simulink model "MQIF_Neuron"  (R2024b)
settings: Solver=ode1  StartTime=0.0  StopTime=10  FixedStep=1e-4  RelTol=1e-3
undefined symbols (not defined in the file): Vus0
settings Model: Creator=Serious Chimp  LastModifiedBy=31194
settings SolverCC: EnableFixedStepZeroCrossing=on
settings RTWCC: GPUComputeCapability=3.5

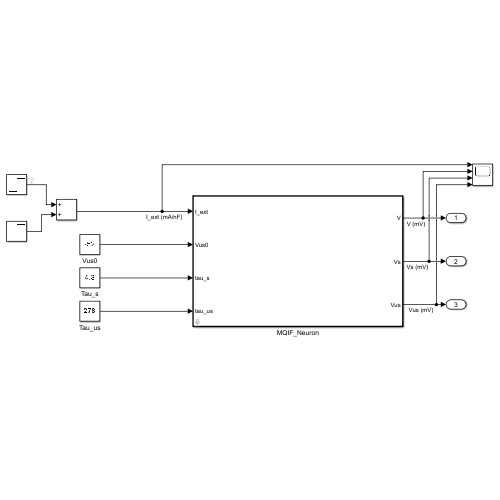
[thumbnail: Simulink's stored preview of the top-level diagram]
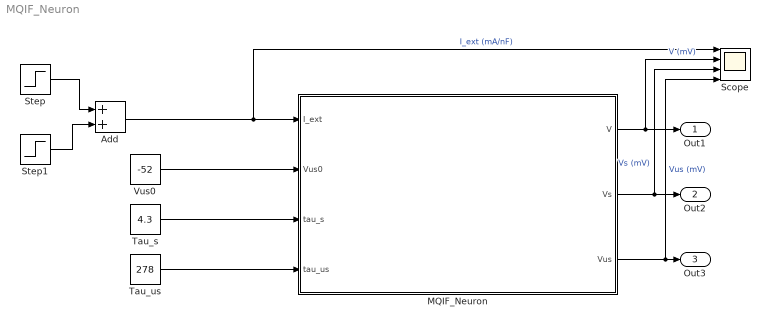
== system MQIF_Neuron ==
  Add : Sum
  MQIF_Neuron : Subsystem  TreatAsAtomicUnit=on  mask{V0=-52, Vs0=-50, V_threshold=20, V_reset=-45, Vs_reset=7.5, delta_Vus=1.7, g_f=1.0, g_s=0.5, g_us=0.015, C=0.82}
      mask prompts: V0 "Equilibrium V0"; Vs0 "Equilibrium Vs0"; V_threshold "Threshold for Spike, V_thresh"; V_reset "After-spike Reset Votlage, V_r"; Vs_reset "After-spike Reset Vs, Vs_r"; delta_Vus "Vus After-spike Memory, delta_Vus"; g_f "I Conductance, g_f"; g_s "I_us Conductance, g_s"; g_us "I_us Conductance, g_us"; C "Capacitance, C"
      mask DialogControl NeuronStateVariables Prompt: Parameters
  Scope : Scope  NumInputPorts=4
  Step : Step  After=5  SampleTime=0
  Step1 : Step  Time=0  After=0  SampleTime=0
  Tau_s : Constant  Value=4.3
  Tau_us : Constant  Value=278
  Vus0 : Constant  Value=-52
  Out1 : Outport
  Out2 : Outport  Port=2
  Out3 : Outport  Port=3
  wires:
  Add/1 -> Scope/1, MQIF_Neuron/1(I_ext)  "I_ext (mA/nF)"
  MQIF_Neuron/1(V) -> Scope/2, Out1/1  "V (mV)"
  MQIF_Neuron/2(Vs) -> Scope/3, Out2/1  "Vs (mV)"
  MQIF_Neuron/3(Vus) -> Scope/4, Out3/1  "Vus (mV)"
  Vus0/1 -> MQIF_Neuron/2(Vus0)
  Tau_s/1 -> MQIF_Neuron/3(tau_s)
  Tau_us/1 -> MQIF_Neuron/4(tau_us)
  Step/1 -> Add/1
  Step1/1 -> Add/2

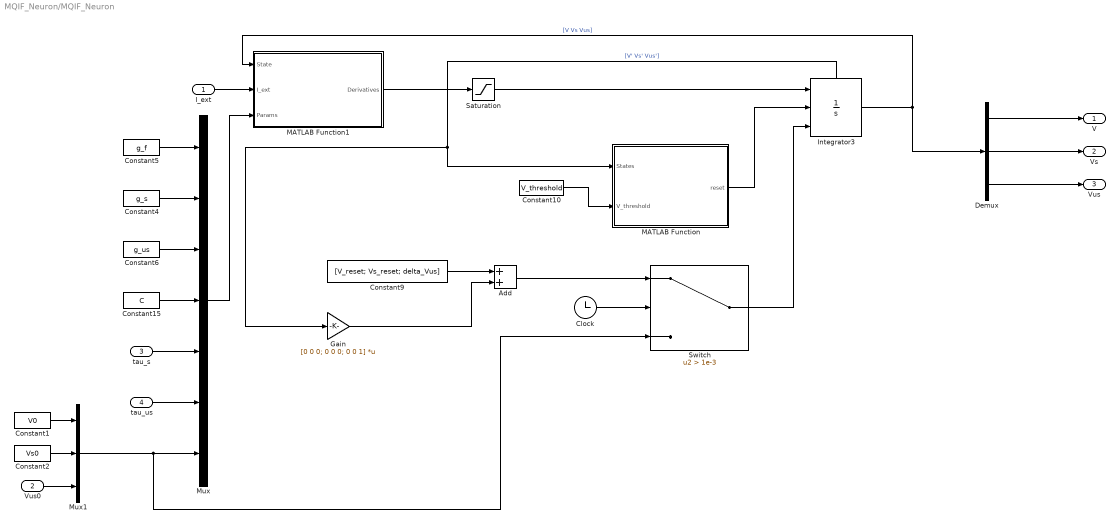
== system MQIF_Neuron/MQIF_Neuron ==
  I_ext : Inport
  Vus0 : Inport  Port=2
  tau_s : Inport  Port=3
  tau_us : Inport  Port=4
  Add : Sum
  Clock : Clock
  Constant1 : Constant  Value=V0
  Constant10 : Constant  Value=V_threshold
  Constant15 : Constant  Value=C
  Constant2 : Constant  Value=Vs0
  Constant4 : Constant  Value=g_s
  Constant5 : Constant  Value=g_f
  Constant6 : Constant  Value=g_us
  Constant9 : Constant  Value=[V_reset; Vs_reset; delta_Vus]
  Demux : Demux  Outputs=3
  Gain : Gain  Gain=[0 0 0; 0 0 0; 0 0 1]  Multiplication=Matrix(K*u) (u vector)
  Integrator3 : Integrator  ExternalReset=rising  InitialConditionSource=external  InitialCondition=[V0 Vs0 Vus0]  LimitOutput=on  UpperSaturationLimit=[30; 10; inf]  LowerSaturationLimit=[-100; -100; -100]  ShowStatePort=on
  MATLAB Function : MATLAB Function  TreatAsAtomicUnit=on
  MATLAB Function1 : MATLAB Function  TreatAsAtomicUnit=on
  Mux : Mux  Inputs=7
  Mux1 : Mux  Inputs=3
  Saturation : Saturate  UpperLimit=10^4  LowerLimit=-10^4
  Switch : Switch  Criteria=u2 > Threshold  Threshold=1e-3  SaturateOnIntegerOverflow=off  InputSameDT=off
  V : Outport
  Vs : Outport  Port=2
  Vus : Outport  Port=3
  wires:
  I_ext/1 -> MATLAB Function1/2(I_ext)
  Constant1/1 -> Mux1/1
  Vus0/1 -> Mux1/3
  Constant5/1 -> Mux/1
  Constant4/1 -> Mux/2
  Constant6/1 -> Mux/3
  Constant15/1 -> Mux/4
  Mux/1 -> MATLAB Function1/3(Params)
  tau_s/1 -> Mux/5
  tau_us/1 -> Mux/6
  Constant10/1 -> MATLAB Function/2(V_threshold)
  Integrator3/1 -> MATLAB Function1/1(State), Demux/1  "[V Vs Vus]"
  Demux/1 -> V/1
  Demux/2 -> Vs/1
  Demux/3 -> Vus/1
  MATLAB Function/1(reset) -> Integrator3/2
  Clock/1 -> Switch/2
  Constant9/1 -> Add/1
  Switch/1 -> Integrator3/3
  Gain/1 -> Add/2
  MATLAB Function1/1(Derivatives) -> Saturation/1
  Add/1 -> Switch/1
  Integrator3/State -> Gain/1, MATLAB Function/1(States)  "[V' Vs' Vus']"
  Mux1/1 -> Switch/3, Mux/7
  Constant2/1 -> Mux1/2
  Saturation/1 -> Integrator3/1

== matlab function MQIF_Neuron/MATLAB Function1 ==
  data: State input; Derivatives output; I_ext input; Params input
function Derivatives = ODE(State, I_ext, Params)
    V = State(1);
    Vs = State(2);
    Vus = State(3);

    g_f = Params(1);
    g_s = Params(2);
    g_us = Params(3);
    C = Params(4);
    tau_s = Params(5);
    tau_us = Params(6);
    V0 = Params(7);
    Vs0 = Params(8);
    Vus0 = Params(9);

    
    V_dot = 250*((I_ext + g_f*((V-V0)^2) - g_s*((Vs-Vs0)^2) - g_us*((Vus-Vus0)^2)) / C);
    Vs_dot = 250*((V - Vs) / tau_s);
    Vus_dot = 250*((V - Vus) / tau_us);

    Derivatives = [V_dot; Vs_dot; Vus_dot];
end

== matlab function MQIF_Neuron/MATLAB Function ==
  data: States input; reset output; V_threshold input
function reset = ResetTrigger(States, V_threshold)

V = States(1);

reset = (V > V_threshold);

end
